simulink model "ss_topology"  (R2020a)
settings: Solver=ode23tb  StartTime=0.0  StopTime=0.0001  MaxStep=1e-8  RelTol=1e-7
undefined symbols (not defined in the file): Cp, Cs, f, Lp, Ls, M, Rc, Rp, Rs, V
libraries: powerlib x8, powerlib_meascontrol x5, eePowerMeasurement x2
settings Model: Creator=Vitor  LastModifiedBy=Vitor
settings DebuggingCC: UnconnectedInputMsg=none  UnconnectedOutputMsg=none  UnconnectedLineMsg=none

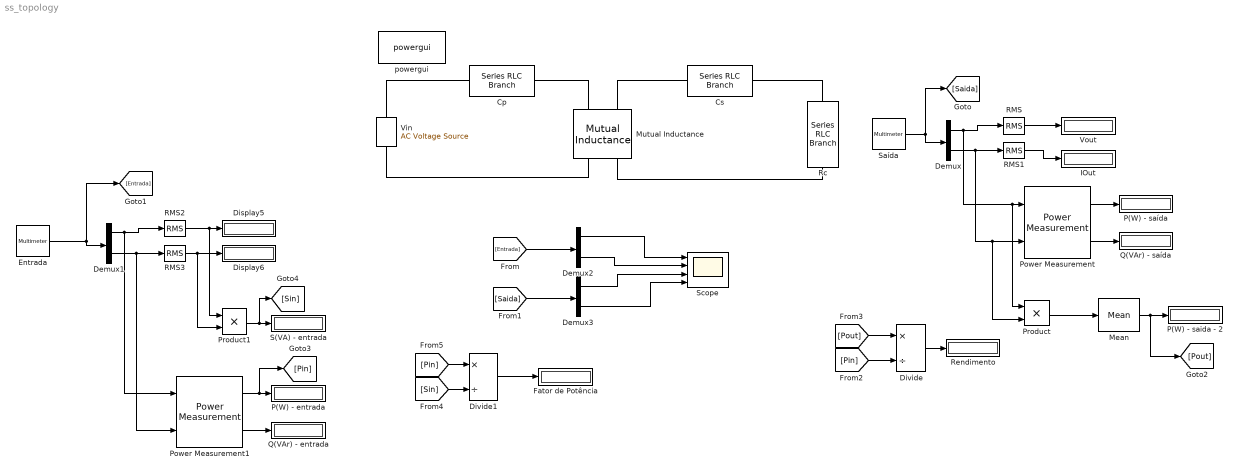
== system ss_topology ==
  Cp : powerlib/Elements/Series RLC Branch  LConnTagsString=__new0  RConnTagsString=__new0  BranchType=C  Resistance=1  Inductance=1e-3  SetiL0=off  InitialCurrent=0  Capacitance=Cp  Setx0=off  InitialVoltage=0  Measurements=Branch current
  Cs : powerlib/Elements/Series RLC Branch  LConnTagsString=__new0  RConnTagsString=__new0  BranchType=C  Resistance=1  Inductance=1e-3  SetiL0=off  InitialCurrent=0  Capacitance=Cs  Setx0=off  InitialVoltage=0  Measurements=None
  Demux{,1..3} (4 alike) : Demux  Outputs=2
  Display5 : Display
  Display6 : Display
  Divide : Product  Inputs=*/  RndMeth=Zero  SaturateOnIntegerOverflow=on
  Divide1 : Product  Inputs=*/  RndMeth=Zero  SaturateOnIntegerOverflow=on
  Entrada : powerlib/Measurements/Multimeter  PhasorSimulation=off  OutputType=Complex  sel=[2 3]  L=4  Gain=[1 1]  yselected={'Usrc: Vin','Ib: Cp'};  PSBOutputType=1  PSBequivalent=0  AxesSetting=[0,0.1,-100,100]  Display=0  SavedBlockNames=-11
  Fator de Potência : Display
  IOut : Display
  Mean : powerlib_meascontrol/Measurements/Mean  Freq=f  Vinit=0  Ts=0
  Mutual Inductance : powerlib/Elements/Mutual Inductance  LConnTagsString=a|b  RConnTagsString=A|B  TypeOfMutual=Two or three windings with equal mutual terms  NumberOfWindings=3  SelfImpedance1=[Rp Lp]  SelfImpedance2=[Rs Ls]  ThreeWindings=off  SelfImpedance3=[ 1.1 1.1e-03]  MutualImpedance=[0 M]  InductanceMatrix="[1.0 0.9  0.9 ;  0.9 1.0  0.9;  0.9 0.9 1.0 ] * 1e-3"  ResistanceMatrix="[1.0 0.9  0.9 ;  0.9 1.0  0.9;  0.9 0.9 1.0 ]"  Measurements=None
      settings: AttributesFormatString=\n  SourceProductBaseCode=PS
  P(W) - entrada : Display
  P(W) - saida - 2 : Display
  P(W) - saída : Display
  Power Measurement : eePowerMeasurement/Power Measurement  LabelModeActiveChoice=Continuous  F=f  K=1  Ts=0
      settings: SourceProductBaseCode=PS
  Power Measurement1 : eePowerMeasurement/Power Measurement  LabelModeActiveChoice=Continuous  F=f  K=1  Ts=0
      settings: SourceProductBaseCode=PS
  Product : Product
  Product1 : Product
  Q(VAr) - entrada : Display
  Q(VAr) - saída : Display
  RMS{,1..3} (4 alike) : powerlib_meascontrol/Measurements/RMS  TrueRMS=on  Freq=f  RMSInit=0  Ts=0
  Rc : powerlib/Elements/Series RLC Branch  LConnTagsString=__new0  RConnTagsString=__new0  BranchType=R  Resistance=Rc  Inductance=1e-3  SetiL0=off  InitialCurrent=0  Capacitance=Cs  Setx0=off  InitialVoltage=0  Measurements=Branch voltage and current
  Rendimento : Display
  S(VA) - entrada : Display
  Saída : powerlib/Measurements/Multimeter  PhasorSimulation=off  OutputType=Complex  sel=[1 4]  L=4  Gain=[1 1]  yselected={'Ub: Rc','Ib: Rc'};  PSBOutputType=1  PSBequivalent=0  AxesSetting=[0,0.1,-100,100]  Display=0  SavedBlockNames=-11
  Scope : Scope  NumInputPorts=4
  Vin : powerlib/Electrical Sources/AC Voltage Source  Amplitude=V  Phase=0  Frequency=f  SampleTime=0  Measurements=Voltage  BusType=swing  Pref=10e3  Qref=0  Qmin=-inf  Qmax=+inf
  Vout : Display
  powergui : powerlib/powergui  Priority=1  SimulationMode=Continuous  SampleTime=50e-6  frequency=60  Iterations=50  frequencyindice=50000  Pbase=100e6  ErrMax=1e-4  UnitsV=kV  UnitsW=MW  buscounter=0  FunctionMessages=off  echomessages=off  EnableUseOfTLC=off  CurrentSourceSwitches=off  DisableSnubberDevices=off  DisableRonSwitches=off  DisableVfSwitches=off  DisplayEquations=off  AutomaticDiscreteSolvers=off  SolverType=Tustin/Backward Euler (TBE)  Interpol=off  ExternalGateDelay=off  methode=off  Ts=100  x0status=blocks  SPID=on  SwTol=0  HookPort=off  NonlinearTolerance=1e-4  nMaxIteration=100  ContinueOnMaxIteration=off  RestoreLinks=warning  ResistiveCurrentMeasurement=off  Frange=[0:2:500]  Ylog=off  Xlog=on  ShowGrid=off  save=off  variable=ZData  structure=0  ZoomFFT=off  StartTime=0.0  cycles=1  DisplayStyle=1  fundamental=60  FreqAxis=off  MaxFrequency=1000  frequencyindicesteady=1  RmsSteady=1  display=off
  wires:
  Saída/1 -> [Saida], Demux/1
  Demux/1 -> Product/1, Power Measurement/1, RMS/1
  Demux/2 -> Power Measurement/2, Product/2, RMS1/1
  RMS/1 -> Vout/1
  RMS1/1 -> IOut/1
  Power Measurement/1 -> P(W) - saída/1
  Power Measurement/2 -> Q(VAr) - saída/1
  Product/1 -> Mean/1
  Mean/1 -> [Pout], P(W) - saida - 2/1
  Demux1/2 -> Power Measurement1/2, RMS3/1
  RMS2/1 -> Product1/1, Display5/1
  Power Measurement1/1 -> [Pin], P(W) - entrada/1
  Power Measurement1/2 -> Q(VAr) - entrada/1
  Entrada/1 -> [Entrada], Demux1/1
  RMS3/1 -> Display6/1, Product1/2
  Demux1/1 -> Power Measurement1/1, RMS2/1
  Product1/1 -> [Sin], S(VA) - entrada/1
  [Entrada] -> Demux2/1
  [Saida] -> Demux3/1
  Demux2/2 -> Scope/2
  Demux2/1 -> Scope/1
  Demux3/1 -> Scope/3
  Demux3/2 -> Scope/4
  Divide/1 -> Rendimento/1
  [Pout] -> Divide/1
  [Pin] -> Divide/2
  Divide1/1 -> Fator de Potência/1
  [Sin] -> Divide1/2
  [Pin] -> Divide1/1
  connections:
  Cp/RConn1 -- Mutual Inductance/LConn1
  Vin/RConn1 -- Cp/LConn1
  Vin/LConn1 -- Mutual Inductance/RConn1
  Cs/LConn1 -- Mutual Inductance/LConn2
  Cs/RConn1 -- Rc/LConn1
  Mutual Inductance/RConn2 -- Rc/RConn1
